simulink model "takeoffANDlandingV5_23b"  (R2023b)
settings: Solver=ode4  StartTime=0.0  StopTime=450  FixedStep=0.001  RelTol=1e-3
values from neighbouring files (symbols this model uses):
  a0 = 340.294    [basedata.m]    (also in basedata.mat; control_design.mat; landing_init.m; landing_plan.mat)
  b_ref = 2.0    (= 2)    [basedata.m]    (also in basedata.mat; control_design.mat; landing_init.m; landing_plan.mat)
  c_gear = [0.8e4, 1.4e4, 1.4e4]    [basedata.m]    (also in basedata.mat = [8000 14000 14000]; control_design.mat = [8000 14000 14000]; landing_init.m; landing_plan.mat = [8000 14000 14000])
  c_lat = [1.4e4, 2.2e4, 2.2e4]    [basedata.m]    (also in basedata.mat = [14000 22000 22000]; control_design.mat = [14000 22000 22000]; landing_init.m; landing_plan.mat = [14000 22000 22000])
  c_ref = 0.9    [basedata.m]    (also in basedata.mat; control_design.mat; landing_init.m; landing_plan.mat)
  c_roll = [0.020, 0.018, 0.018]    [basedata.m]    (also in basedata.mat = [0.02 0.018 0.018]; control_design.mat = [0.02 0.018 0.018]; landing_init.m; landing_plan.mat = [0.02 0.018 0.018])
  CD0 = 0.045    [basedata.m]    (also in basedata.mat; canshujisuan.m; control_design.mat; landing_init.m)
  CL0 = 0.083    [basedata.m]    (also in basedata.mat; control_design.mat; landing_init.m; landing_plan.mat)
  CLa = 3.80    (= 3.8)    [basedata.m]    (also in basedata.mat; canshujisuan.m = 2.5; control_design.mat; landing_init.m)
  Clb = -0.08    [basedata.m]    (also in basedata.mat; control_design.mat; landing_init.m; landing_plan.mat)
  Clda = -0.20    (= -0.2)    [basedata.m]    (also in basedata.mat; control_design.mat; landing_init.m; landing_plan.mat)
  CLde = 0.28    [basedata.m]    (also in basedata.mat; control_design.mat; landing_init.m; landing_plan.mat)
  Clp = -0.70    (= -0.7)    [basedata.m]    (also in basedata.mat; control_design.mat; landing_init.m; landing_plan.mat)
  CLq = 4.50    (= 4.5)    [basedata.m]    (also in basedata.mat; canshujisuan.m = 3; control_design.mat; landing_init.m)
  Clr = 0.08    [basedata.m]    (also in basedata.mat; control_design.mat; landing_init.m; landing_plan.mat)
  Cm0 = 0.060    (= 0.06)    [basedata.m]    (also in basedata.mat; control_design.mat; landing_init.m; landing_plan.mat)
  Cma = -0.80    (= -0.8)    [basedata.m]    (also in basedata.mat; control_design.mat; landing_init.m; landing_plan.mat)
  Cmde = -0.90    (= -0.9)    [basedata.m]    (also in basedata.mat; control_design.mat; landing_init.m; landing_plan.mat)
  Cmq = -18.0    (= -18)    [basedata.m]    (also in basedata.mat; control_design.mat; landing_init.m; landing_plan.mat)
  Cnb = 0.25    [basedata.m]    (also in basedata.mat; control_design.mat; landing_init.m; landing_plan.mat)
  Cndr = -0.15    [basedata.m]    (also in basedata.mat; control_design.mat; landing_init.m; landing_plan.mat)
  Cnp = -0.04    [basedata.m]    (also in basedata.mat; control_design.mat; landing_init.m; landing_plan.mat)
  Cnr = -0.45    [basedata.m]    (also in basedata.mat; control_design.mat; landing_init.m; landing_plan.mat)
  CSb = -0.70    (= -0.7)    [basedata.m]    (also in basedata.mat; control_design.mat; landing_init.m; landing_plan.mat)
  CSdr = 0.18    [basedata.m]    (also in basedata.mat; control_design.mat; landing_init.m; landing_plan.mat)
  CSr = 0.12    [basedata.m]    (also in basedata.mat; control_design.mat; landing_init.m; landing_plan.mat)
  D = 0.5 * rho0 * V^2 * S_ref * CD_current    [canshujisuan.m]
  D0 = 1400    [basedata.m]    (also in basedata.mat; control_design.mat = 800; landing.m; landing_init.m)
  da_max = 25    [basedata.m]    (also in basedata.mat; control_design.mat; landing_init.m; landing_plan.mat)
  da_min = -da_max    (= -25)    [basedata.m]    (also in basedata.mat; control_design.mat; landing_init.m; landing_plan.mat)
  de_max = 25    [basedata.m]    (also in basedata.mat; control_design.mat; landing_init.m; landing_plan.mat)
  de_min = -de_max    (= -25)    [basedata.m]    (also in basedata.mat; control_design.mat; landing_init.m; landing_plan.mat)
  DH = pi / 180    (= 0.0174532925199)    [basedata.m]    (also in basedata.mat; control_design.mat; landing_init.m; landing_plan.mat)
  dr_max = 25    [basedata.m]    (also in basedata.mat; control_design.mat; landing_init.m; landing_plan.mat)
  dr_min = -dr_max    (= -25)    [basedata.m]    (also in basedata.mat; control_design.mat; landing_init.m; landing_plan.mat)
  g = 9.80665    [basedata.m]    (also in basedata.mat; canshujisuan.m; control_design.mat; landing_init.m)
  ground_z = 0.0    (= 0)    [basedata.m]    (also in basedata.mat; control_design.mat; landing_init.m; landing_plan.mat)
  H_B = 132.622761894    [basedata.mat]    (also in landing_trajectory.m = H_R - R * cos(a1); landingplan.mat)
  H_C = 72.1000994005    [basedata.mat]    (also in landing_trajectory.m = H_R - R * cos(a2); landingplan.mat)
  H_climb_complete = 1000    [control_design.mat]    (also in landing.m; landing_init.m; landing_plan.mat; landingplan.mat)
  H_entry = 1000    [basedata.mat]    (also in landing_trajectory.m; landingplan.mat)
  H_exp = 20    [basedata.mat]    (also in landing_trajectory.m; landingplan.mat)
  HD = 180 / pi    (= 57.2957795131)    [basedata.m]    (also in basedata.mat; control_design.mat; landing_init.m; landing_plan.mat)
  I = [ Ixx, -Ixy, -Ixz ... (first row only)    [basedata.m]    (also in basedata.mat = [120  0  0; 0  480  0; 0  0  520]; control_design.mat = [120  0  0; 0  480  0; 0  0  520]; landing_init.m; landing_plan.mat = [120  0  0; 0  480  0; 0  0  520])
  K = 0.12    [basedata.m]    (also in basedata.mat; canshujisuan.m = 0.08; control_design.mat; landing_init.m)
  K_alpha = 7.5375    [basedata.mat]    (also in control_design.m = (((wd_pitch^2)-a24))/(2*kesi_pitch*wd_pitch); control_design.mat; controller.m = 5; landingplan.mat)
  k_gear = [1.0e5, 3.0e5, 3.0e5]    [basedata.m]    (also in basedata.mat = [100000 300000 300000]; control_design.mat = [100000 300000 300000]; landing_init.m; landing_plan.mat = [100000 300000 300000])
  Kn_pitch = -0.120095403309    [basedata.mat]    (also in control_design.m = -(2.2*g*(wd_pitch)^2)/(Tr*(((wd_pitch)^2)-a24)*V_control*a34; control_design.mat; controller.m = (2.2*wd^2*g)/(Tr*(wd^2-a24)*V_test*a34); landingplan.mat)
  Kw_pitch = -0.483749055178    [basedata.mat]    (also in control_design.m = -2*kesi_pitch*wd_pitch/a25; control_design.mat; controller.m = -(2*zeta*wd) / a25; landingplan.mat)
  m = 600.0    (= 600)    [basedata.m]    (also in basedata.mat; canshujisuan.m; control_design.mat; landing_init.m)
  mu_brake = [0.0, 0.55, 0.55]    [basedata.m]    (also in basedata.mat = [0 0.55 0.55]; control_design.mat = [0 0.55 0.55]; landing_init.m; landing_plan.mat = [0 0.55 0.55])
  phi0 = 0    [control_design.mat]    (also in landing.m; landing_init.m; landing_init.mat; landing_plan.mat)
  psi0 = 0    [control_design.mat]    (also in landing.m; landing_init.m; landing_init.mat; landing_plan.mat)
  r_left_b = r_gear_b(:,2)    [basedata.m]    (also in basedata.mat = [-0.333333333333 -0.8 0.65]; control_design.mat = [-0.333333333333 -0.8 0.65]; landing_init.m; landing_plan.mat = [-0.333333333333 -0.8 0.65])
  r_nose_b = r_gear_b(:,1)    [basedata.m]    (also in basedata.mat = [2 0 0.65]; control_design.mat = [2 0 0.65]; landing_init.m; landing_plan.mat = [2 0 0.65])
  r_right_b = r_gear_b(:,3)    [basedata.m]    (also in basedata.mat = [-0.333333333333 0.8 0.65]; control_design.mat = [-0.333333333333 0.8 0.65]; landing_init.m; landing_plan.mat = [-0.333333333333 0.8 0.65])
  rho0 = 1.225    [basedata.m]    (also in basedata.mat; canshujisuan.m; control_design.mat; landing_init.m)
  S_ref = 1.2    [basedata.m]    (also in basedata.mat; canshujisuan.m; control_design.mat; landing_init.m)
  theta0 = 0    [control_design.mat]    (also in landing.m; landing_init.m; landing_init.mat = 0.0523598775598; landing_plan.mat = 0.0523560209424)
  u0_b = 0    [control_design.mat]    (also in landing.m = 128; landing_init.m = 128; landing_init.mat = 100; landing_plan.mat = 128)
  v0_b = 0    [control_design.mat]    (also in landing.m; landing_init.m; landing_init.mat; landing_plan.mat)
  V_app = 128.516392565    [basedata.mat]    (also in landing_trajectory.m = 1.4 * Vs; landingplan.mat)
  V_cruise = 200    [basedata.m]
  v_eps = 0.20    (= 0.2)    [basedata.m]    (also in basedata.mat; control_design.mat; landing_init.m; landing_plan.mat)
  V_flare = V_shallow    [landing_trajectory.m]
  V_min = 3    [control_design.mat]    (also in landing.m; landing_init.m; landing_plan.mat; landingplan.mat)
  V_shallow = 110.156907913    [basedata.mat]    (also in landing_trajectory.m = 1.2 * Vs; landingplan.mat)
  w0_b = 0    [control_design.mat]    (also in landing.m; landing_init.m; landing_init.mat; landing_plan.mat)
  wheel_radius = 0.18    [basedata.m]    (also in basedata.mat; control_design.mat; landing_init.m; landing_plan.mat)
  WOW_on = 0.000    (= 0)    [basedata.m]    (also in basedata.mat; control_design.mat; landing_init.m; landing_plan.mat)
  Xg0 = 0    [control_design.mat]    (also in landing.m = -12000; landing_init.m = -12000; landing_init.mat = -8000; landing_plan.mat = -12000)
  Yg0 = 3    [control_design.mat]    (also in landing.m = 0; landing_init.m = 0; landing_init.mat = 0; landing_plan.mat = 0)
  Zg0 = ground_z - wheel_radius - r_gear_b(3,1) + static_deflection    [basedata.m]    (also in basedata.mat = -0.8215943; control_design.mat = -0.8215943; landing.m = -1000; landing_init.m = -1000)
undefined symbols (not defined in the file or in its folder): H_start, I_xz, I_yz, Ix_Iy, Iy_Iz, Iz_Ix, X_landing_start
libraries: simulink x54, matrix_library x19
(part 4 of 4)

== matlab function takeoffANDlandingV5_23b/Guidance/降落阶段/MATLAB Function ==
  settings: updateMethod=DISCRETE  sampleTime=0.001
  data: gamma_cmd output; Flight_Phase input; H_cmd output; X input; h_AGL input; Vg input
 function [gamma_cmd,H_cmd] = landing_longitudinal_guidance(Flight_Phase, X, h_AGL, Vg)
%#codegen

gamma1 = -0.125844364414799;   % 陡下滑角
gamma2 = -0.0261780104712042;  % 浅下滑角

R_round = 8000.0;

L_capture = 600.0;   % 7/8阶段下滑角过渡距离，m
L_shallow = 500.0;   % 10阶段过渡距离，m
L_flare   = 400.0;   % 11阶段拉平过渡距离，m

V_sink_td = 0.3;     % 接地下沉率，m/s

persistent initialized
persistent last_phase
persistent X_prev H_prev gamma_prev
persistent X_enter H_enter gamma_enter
persistent XR HR

if isempty(initialized)
    initialized = true;

    last_phase = Flight_Phase;

    X_prev = X;
    H_prev = h_AGL;
    gamma_prev = 0.0;

    X_enter = X;
    H_enter = h_AGL;
    gamma_enter = 0.0;

    XR = X;
    HR = h_AGL + R_round;
end

dX = X - X_prev;
if dX < 0.0
    dX = 0.0;
end

% 阶段切换时锁存上一阶段的输出，而不是重新用固定边界
if Flight_Phase ~= last_phase
    X_enter = X;
    H_enter = H_prev;
    gamma_enter = gamma_prev;

    if Flight_Phase == 10
        XR = X_enter - R_round * sin(gamma_enter);
        HR = H_enter + R_round * cos(gamma_enter);
    end

    last_phase = Flight_Phase;
    dX = 0.0;
end

if Flight_Phase == 10
    dx = X - XR;
    rad = R_round^2 - dx^2;

    if rad < 1e-6
        rad = 1e-6;
    end

    H_cmd = HR - sqrt(rad);
    gamma_cmd = atan(dx / sqrt(rad));

else
    if Flight_Phase == 6
        gamma_target = 0.0;
        L_use = L_capture;

    elseif Flight_Phase == 7 || Flight_Phase == 8||Flight_Phase==9
        gamma_target = gamma1;
        L_use = L_capture;

    elseif Flight_Phase == 11
        gamma_target = gamma2;
        L_use = L_shallow;

    elseif Flight_Phase == 12
        V_use = max(Vg, 1.0);
        s = -V_sink_td / V_use;
        s = min(max(s, -1.0), 1.0);

        gamma_target = asin(s);
        L_use = L_flare;

    else
        gamma_target = 0.0;
        L_use = L_capture;
    end

    alpha = 1.0 - exp(-dX / max(L_use, 1.0));

    gamma_cmd = gamma_prev + alpha * (gamma_target - gamma_prev);
    H_cmd = H_prev + tan(gamma_cmd) * dX;

    if Flight_Phase == 12 && H_cmd < 0.0
        H_cmd = 0.0;
        gamma_cmd = 0.0;
    end
end

X_prev = X;
H_prev = H_cmd;
gamma_prev = gamma_cmd;

== matlab function takeoffANDlandingV5_23b/6DOF-MODEL/动力学/height/MATLAB Function1 ==
  data: phi input; R_bg output; theta input; psi input
function R_bg = ground2body(phi, theta, psi)
T1 = [cos(psi), sin(psi), 0;
     -sin(psi), cos(psi), 0;
      0, 0, 1];
T2 = [cos(theta), 0, -sin(theta);
       0, 1, 0;
      sin(theta), 0, cos(theta)];
T3 = [1, 0, 0;
      0, cos(phi), sin(phi);
      0, -sin(phi), cos(phi)];
R_bg = T3 * T2 * T1;

== stateflow chart takeoffANDlandingV5_23b/Flight Phase Manager/Phase Logic ==
  state Takeoff_Mode
    state Ground_Roll
      en: Flight_Phase = 1;
    state Rotation
      en: Flight_Phase = 2;
    state Liftoff
      en: Flight_Phase = 3;
    state Initial_Climb
      en: Flight_Phase = 4;
    state Climb_Complete
      en: Flight_Phase = 5;
    (default) -> Ground_Roll
    Rotation -> Liftoff : [airborne == true]
    Ground_Roll -> Rotation : [reach_VR==true]
    Liftoff -> Initial_Climb : [safe_climb == true]
    Initial_Climb -> Climb_Complete : [in_cruise==true]
  state Landing_Mode
    state Trajectory_Capture_yaw
      en: Flight_Phase = 7;
    state Trajectory_Capture_compelet
      en: Flight_Phase = 8;
    state Steep_Glide
      en: Flight_Phase = 9;
    state Round_Flare
      en: Flight_Phase =10;
    state Approach
      en: Flight_Phase = 6;
    state Roll_out
      en: Flight_Phase = 14;
    state Touchdown
      en: Flight_Phase = 13;
    state Flare
      en: Flight_Phase = 12;
    state Shallow_Glide
      en: Flight_Phase = 11;
    (default) -> Approach
    Trajectory_Capture_yaw -> Trajectory_Capture_compelet : [pitchcaptrue==true]
    Steep_Glide -> Round_Flare : [in_round==true]
    Approach -> Trajectory_Capture_yaw : [yawcapture==true]
    Trajectory_Capture_compelet -> Steep_Glide : [in_steep == true]
    Round_Flare -> Shallow_Glide : [Slight_decline==true]
    Flare -> Touchdown : [touch_ground == true]
    Touchdown -> Roll_out : [in_ground==true]
    Shallow_Glide -> Flare : [in_Flare==true]
  (junction 38) -> Takeoff_Mode [order 1] : [Task_Mode == 1]{Flight_Phase = 0;}
  (default) -> (junction 38)
  (junction 38) -> Landing_Mode [order 2] : {Flight_Phase = 0;}
  Takeoff_Mode -> Landing_Mode : [Task_Mode == 2]
  data: reach_VR input size=1; airborne input size=1; safe_climb input size=1; in_cruise input; Task_Mode input size=1; yawcapture input; pitchcaptrue input; in_steep input; in_round input; Slight_decline input; in_Flare input; touch_ground input; in_ground input; Flight_Phase output uint8 size=1 =0

== matlab function takeoffANDlandingV5_23b/controller1/4_Power&V_Ctrl/MATLAB Function2 ==
  data: Vel_g input; dv_err output; axyz input
function dv_err = dv_cal(Vel_g,axyz)
%#codegen

% k_theta = Att_g(1)*pi/180;
% psi = Att_g(2)*pi/180;
% gama = Att_g(3)*pi/180;
% 
% Cg_b = Mx(gama)*Mz(k_theta)*My(psi);
% Cb_g = Cg_b';
vx = Vel_g(1);
vy = Vel_g(2);
vz = Vel_g(3);

ax = axyz(1);
ay = axyz(2);
az = axyz(3);

dv_err = (vx*ax + vy*ay + vz*az)/sqrt(vx^2 + vy^2 + vz^2);
% dv_err = (vx*ax + vz*az)/sqrt(vx^2 + vz^2);
if isnan(dv_err) == 1 
    dv_err = 0;
end

== matlab function takeoffANDlandingV5_23b/6DOF-MODEL/动力学/起落架模型/纵向力/Subsystem/MATLAB Function ==
  data: phi input; R_bg output; theta input; psi input
function R_bg = ground2body(phi, theta, psi)
T1 = [cos(psi), sin(psi), 0;
     -sin(psi), cos(psi), 0;
      0, 0, 1];
T2 = [cos(theta), 0, -sin(theta);
       0, 1, 0;
      sin(theta), 0, cos(theta)];
T3 = [1, 0, 0;
      0, cos(phi), sin(phi);
      0, -sin(phi), cos(phi)];
R_bg = T3 * T2 * T1;

== matlab function takeoffANDlandingV5_23b/6DOF-MODEL/动力学/起落架模型/纵向力/Subsystem/主轮滚动方向向量 ==
  data: Cbg input; eg_long output; eb_long input
function eg_long = project_long(Cbg, eb_long)

e_z = [0; 0; 1];              % 前-右-下坐标系：Z 轴向下
P_g = eye(3) - e_z*e_z.';     % 投影到地面水平面

eg_long = P_g * Cbg * eb_long;

n = norm(eg_long);
if n > 1e-8
    eg_long = eg_long / n;
else
    eg_long = [1; 0; 0];
end

== matlab function takeoffANDlandingV5_23b/6DOF-MODEL/动力学/起落架模型/纵向力/Subsystem/前轮滚动方向向量 ==
  data: Cbg input; eg_long output; eb_long input
function eg_long = project_long(Cbg, eb_long)

e_z = [0; 0; 1];              % 前-右-下坐标系中，Z 轴为下
P_g = eye(3) - e_z*e_z.';     % 投影到地面水平面

eg_long = P_g * Cbg * eb_long;

n = norm(eg_long);
if n > 1e-8
    eg_long = eg_long / n;
else
    eg_long = [1; 0; 0];
end

== matlab function takeoffANDlandingV5_23b/6DOF-MODEL/动力学/起落架模型/起落架三轮质心在地系下位置/MATLAB Function ==
  data: phi input; R_bg output; theta input; psi input
function R_bg = ground2body(phi, theta, psi)
T1 = [cos(psi), sin(psi), 0;
     -sin(psi), cos(psi), 0;
      0, 0, 1];
T2 = [cos(theta), 0, -sin(theta);
       0, 1, 0;
      sin(theta), 0, cos(theta)];
T3 = [1, 0, 0;
      0, cos(phi), sin(phi);
      0, -sin(phi), cos(phi)];
R_bg = T3 * T2 * T1;
